simulink model "SimNL"  (R2024a)
settings: Solver=ode45  StartTime=0.0  StopTime=10.0  RelTol=1e-3  EnableMultiTasking=on
undefined symbols (not defined in the file or in its folder): ParamReels
settings Model: Creator=nazih  LastModifiedBy=Administrator
settings SolverCC: AlgebraicLoopSolver=TrustRegion
settings DataIOCC: LimitDataPoints=on  SaveFormat=Array  SignalLoggingSaveFormat=ModelDataLogs  ReturnWorkspaceOutputs=off
settings OptimizationCC: BlockReduction=off  BooleanDataType=off  LifeSpan=inf
settings DebuggingCC: SaveWithParameterizedLinksMsg=none  UnderspecifiedInitializationDetection=Classic  MergeDetectMultiDrivingBlocksExec=none  SignalResolutionControl=TryResolveAllWithWarning  MultiTaskDSMMsg=warning  MultiTaskCondExecSysMsg=none  UnconnectedInputMsg=warning  UnconnectedOutputMsg=warning  UnconnectedLineMsg=warning  StateNameClashWarn=warning  SFUnexpectedBacktrackingDiag=warning  SFNoUnconditionalDefaultTransitionDiag=warning  SFExecutionAtInitializationDiag=none  ArithmeticOperatorsInVariantConditions=warning
settings HardwareCC: ProdBitPerPointer=32  ProdBitPerSizeT=32  ProdBitPerPtrDiffT=32  ProdLargestAtomicFloat=None  ProdIntDivRoundTo=Undefined  ProdEndianess=Unspecified  ProdWordSize=32  ProdHWDeviceType=32-bit Generic  TargetUnknown=on
settings ModelReferenceCC: PropagateSignalLabelsOutOfModel=off
settings SFSimCC: SimUseLocalCustomCode=off  CustomCodeUndefinedFunction=UseInterfaceOnly
settings RTWCC: RTWUseLocalCustomCode=off  GPUComputeCapability=3.5
settings CodeAppCC: StateflowObjectComments=on
settings GRTTargetCC: TargetLangStandard=C89/C90 (ANSI)  CombineOutputUpdateFcns=off  GRTInterface=on
settings ConfigComp: CovMetricSettings=dw  CovSaveCumulativeToWorkspaceVar=on  CovSaveSingleToWorkspaceVar=on  CovExternalEMLEnable=off

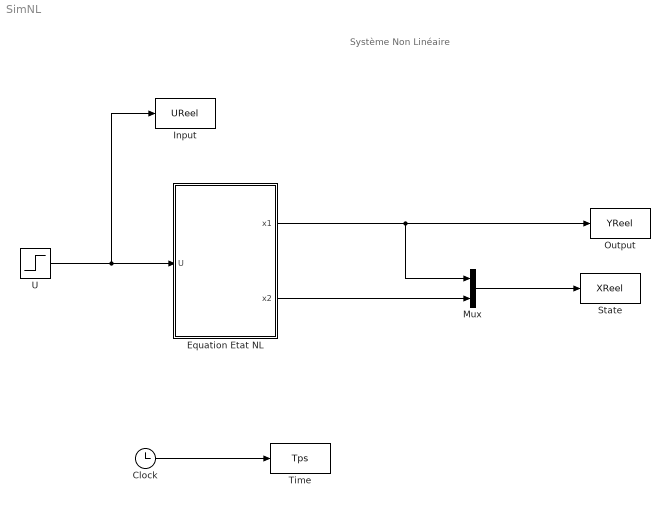
== system SimNL ==
  note: Système Non Linéaire
  Clock : Clock
  Equation Etat NL : Subsystem
  Input : ToWorkspace  VariableName=UReel  SampleTime=ParamReels.Te
  Mux : Mux  Inputs=2
  Output : ToWorkspace  VariableName=YReel  SampleTime=ParamReels.Te
  State : ToWorkspace  VariableName=XReel  SampleTime=ParamReels.Te
  Time : ToWorkspace  VariableName=Tps  SampleTime=ParamReels.Te
  U : Step  Time=4  Before=ParamReels.Equilibre.Ue  After=ParamReels.Equilibre.Ue+1  SampleTime=0
  wires:
  U/1 -> Input/1, Equation Etat NL/1(U)
  Equation Etat NL/2(x2) -> Mux/2
  Equation Etat NL/1(x1) -> Mux/1, Output/1
  Clock/1 -> Time/1
  Mux/1 -> State/1

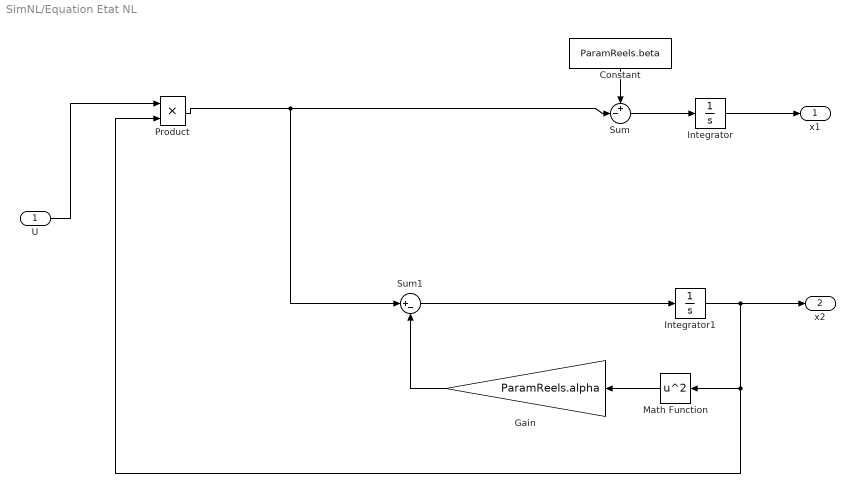
== system SimNL/Equation Etat NL ==
  U : Inport
  Constant : Constant  Value=ParamReels.beta
  Gain : Gain  Gain=ParamReels.alpha  SaturateOnIntegerOverflow=on  OutDataTypeStr=Inherit: Same as input  ParamDataTypeStr=Inherit: Same as input
  Integrator : Integrator  InitialCondition=ParamReels.X0(1,1)
  Integrator1 : Integrator  InitialCondition=ParamReels.X0(2,1)
  Math Function : Math  Operator=square  SignedPower=on
  Product : Product  InputSameDT=on  RndMeth=Zero  SaturateOnIntegerOverflow=on  OutDataTypeStr=Inherit: Same as first input
  Sum : Sum  Inputs=+-|  InputSameDT=on  SaturateOnIntegerOverflow=on  OutDataTypeStr=Inherit: Same as first input
  Sum1 : Sum  Inputs=|+-  InputSameDT=on  SaturateOnIntegerOverflow=on  OutDataTypeStr=Inherit: Same as first input
  x1 : Outport
  x2 : Outport  Port=2
  wires:
  Integrator1/1 -> x2/1, Product/2, Math Function/1
  Integrator/1 -> x1/1
  Sum/1 -> Integrator/1
  Product/1 -> Sum/2, Sum1/1
  U/1 -> Product/1
  Constant/1 -> Sum/1
  Math Function/1 -> Gain/1
  Sum1/1 -> Integrator1/1
  Gain/1 -> Sum1/2
